simulink model "PID"  (R2021b)
settings: Solver=VariableStepAuto  StartTime=0.0  StopTime=inf  RelTol=1e-3
undefined symbols (not defined in the file or in its folder): K, my_password, recipient, sender, sendMail, T
libraries: slpidlib x2, flexy2_lib x1, dspstat3 x1
settings Model: Creator=timon  LastModifiedBy=marekwadinger

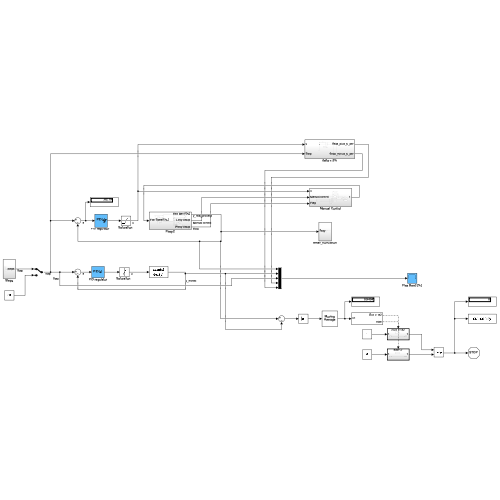
[thumbnail: Simulink's stored preview of the top-level diagram]
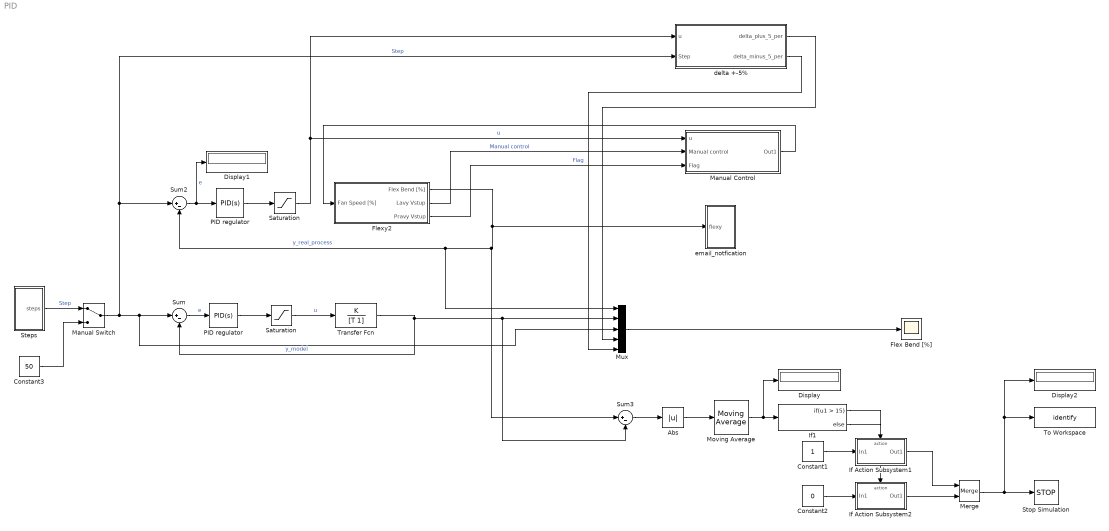
== system PID ==
  Abs : Abs
  Constant1 : Constant
  Constant2 : Constant  Value=0
  Constant3 : Constant  Value=50
  Display : Display
  Display1 : Display
  Display2 : Display
  Flex Bend [%] : Scope
  Flexy2 : Subsystem
  If Action Subsystem1 : Subsystem  TreatAsAtomicUnit=on
  If Action Subsystem2 : Subsystem  TreatAsAtomicUnit=on
  If1 : If  IfExpression=u1 > 15
  Manual Control : Subsystem
  Manual Switch : ManualSwitch
  Merge : Merge
  Moving Average : dspstat3/Moving Average  Method=Sliding window  ForgettingFactorPort=off  SpecifyWindowLength=on  WindowLength=10000  ForgettingFactor=0.9  SimulateUsing=Code generation
  Mux : Mux  Inputs=5
  PID regulator : slpidlib/PID Controller  Controller=PID  Form=Parallel  TimeDomain=Continuous-time  UseExternalTs=off  SampleTime=-1  IntegratorMethod=Forward Euler  FilterMethod=Forward Euler  ControllerParametersSource=internal  P=2.611  I=2.611/0.32485  D=2.611*0.082197  UseFilter=on  N=100  TunerSelectOption=Transfer Function Based (PID Tuner App)  InitialConditionSource=internal  InitialConditionForIntegrator=0  InitialConditionForFilter=0  DifferentiatorICPrevScaledInput=0  ExternalReset=none  TrackingMode=off  Kt=1  LimitOutput=off  SatLimitsSource=internal  UpperSaturationLimit=inf  LowerSaturationLimit=-inf  LinearizeAsGain=on  AntiWindupMode=none  Kb=1  POutMin=[]  POutMax=[]  IOutMin=[]  IOutMax=[]  DOutMin=[]  DOutMax=[]  NOutMin=[]  NOutMax=[]  SumOutMin=[]  SumOutMax=[]  SaturationOutMin=[]  SaturationOutMax=[]  PParamMin=[]  PParamMax=[]  IParamMin=[]  IParamMax=[]  DParamMin=[]  DParamMax=[]  NParamMin=[]  NParamMax=[]  KbParamMin=[]  KbParamMax=[]  KtParamMin=[]  KtParamMax=[]  KbOutMin=[]  KbOutMax=[]  KtOutMin=[]  KtOutMax=[]  IntegratorOutMin=[]  IntegratorOutMax=[]  FilterOutMin=[]  FilterOutMax=[]  SumI1OutMin=[]  SumI1OutMax=[]  SumI2OutMin=[]  SumI2OutMax=[]  SumI3OutMin=[]  SumI3OutMax=[]  SumI4OutMin=[]  SumI4OutMax=[]  SumDOutMin=[]  SumDOutMax=[]  DifferentiatorOutMin=[]  DifferentiatorOutMax=[]  FilterDiffOutCoefMin=[]  FilterDiffOutCoefMax=[]  ReciprocalOutMin=[]  ReciprocalOutMax=[]  SumDenOutMin=[]  SumDenOutMax=[]  SumNumOutMin=[]  SumNumOutMax=[]  DivideOutMin=[]  DivideOutMax=[]  UdiffTsProdOutMin=[]  UdiffTsProdOutMax=[]  NTsProdOutMin=[]  NTsProdOutMax=[]  UintegralTsProdOutMin=[]  UintegralTsProdOutMax=[]  UngainTsProdOutMin=[]  UngainTsProdOutMax=[]  IntegratorContinuousStateAttributes=''  IntegratorStateMustResolveToSignalObject=off  IntegratorRTWStateStorageClass=Auto  FilterContinuousStateAttributes=''  FilterStateMustResolveToSignalObject=off  FilterRTWStateStorageClass=Auto  ParallelPVariant=InternalParameters  IdealPVariant=Disabled  IVariant=InternalParameters  DVariant=InternalParameters  IntegratorVariant=Continuous  SatVariant=Disabled  AWVariant=Passthrough  PCopyVariant=Disabled  TRVariant=Disabled  FdbkBlocksVariant=Forward  IdealPFdbkVariant=Disabled  SatFdbkVariant=Disabled  DerivativeFilterVariant=ContFilter  NVariant=InternalParameters  NCopyVariant=Disabled  FilterICVariant=InternalICsFilter  IntegratorICVariant=InternalICs  ExternalResetVariant=Disabled  TRSumVariant=Passthrough  SumFdbkVariant=Disabled  SumVariant=Sum_PID  TsampFilterVariant=InternalTs  TsampNgainVariant=Passthrough  TsampIntegralVariant=Passthrough  ExternalSaturationOutDataTypeStr=Inherit: Same as second input
  "PID regulator  " : slpidlib/PID Controller  Controller=PID  Form=Parallel  TimeDomain=Continuous-time  UseExternalTs=off  SampleTime=-1  IntegratorMethod=Forward Euler  FilterMethod=Forward Euler  ControllerParametersSource=internal  P=2.611  I=2.611/0.32485  D=2.611*0.082197  UseFilter=on  N=100  TunerSelectOption=Transfer Function Based (PID Tuner App)  InitialConditionSource=internal  InitialConditionForIntegrator=0  InitialConditionForFilter=0  DifferentiatorICPrevScaledInput=0  ExternalReset=none  TrackingMode=off  Kt=1  LimitOutput=on  SatLimitsSource=internal  UpperSaturationLimit=100  LowerSaturationLimit=0  LinearizeAsGain=on  AntiWindupMode=back-calculation  Kb=1  POutMin=[]  POutMax=[]  IOutMin=[]  IOutMax=[]  DOutMin=[]  DOutMax=[]  NOutMin=[]  NOutMax=[]  SumOutMin=[]  SumOutMax=[]  SaturationOutMin=[]  SaturationOutMax=[]  PParamMin=[]  PParamMax=[]  IParamMin=[]  IParamMax=[]  DParamMin=[]  DParamMax=[]  NParamMin=[]  NParamMax=[]  KbParamMin=[]  KbParamMax=[]  KtParamMin=[]  KtParamMax=[]  KbOutMin=[]  KbOutMax=[]  KtOutMin=[]  KtOutMax=[]  IntegratorOutMin=[]  IntegratorOutMax=[]  FilterOutMin=[]  FilterOutMax=[]  SumI1OutMin=[]  SumI1OutMax=[]  SumI2OutMin=[]  SumI2OutMax=[]  SumI3OutMin=[]  SumI3OutMax=[]  SumI4OutMin=[]  SumI4OutMax=[]  SumDOutMin=[]  SumDOutMax=[]  DifferentiatorOutMin=[]  DifferentiatorOutMax=[]  FilterDiffOutCoefMin=[]  FilterDiffOutCoefMax=[]  ReciprocalOutMin=[]  ReciprocalOutMax=[]  SumDenOutMin=[]  SumDenOutMax=[]  SumNumOutMin=[]  SumNumOutMax=[]  DivideOutMin=[]  DivideOutMax=[]  UdiffTsProdOutMin=[]  UdiffTsProdOutMax=[]  NTsProdOutMin=[]  NTsProdOutMax=[]  UintegralTsProdOutMin=[]  UintegralTsProdOutMax=[]  UngainTsProdOutMin=[]  UngainTsProdOutMax=[]  IntegratorContinuousStateAttributes=''  IntegratorStateMustResolveToSignalObject=off  IntegratorRTWStateStorageClass=Auto  FilterContinuousStateAttributes=''  FilterStateMustResolveToSignalObject=off  FilterRTWStateStorageClass=Auto  ParallelPVariant=InternalParameters  IdealPVariant=Disabled  IVariant=InternalParameters  DVariant=InternalParameters  IntegratorVariant=Continuous  SatVariant=Enabled  AWVariant=BackCalculation  PCopyVariant=Disabled  TRVariant=Disabled  FdbkBlocksVariant=Forward  IdealPFdbkVariant=Disabled  SatFdbkVariant=Disabled  DerivativeFilterVariant=ContFilter  NVariant=InternalParameters  NCopyVariant=Disabled  FilterICVariant=InternalICsFilter  IntegratorICVariant=InternalICs  ExternalResetVariant=Disabled  TRSumVariant=Passthrough  SumFdbkVariant=Disabled  SumVariant=Sum_PID  TsampFilterVariant=InternalTs  TsampNgainVariant=Passthrough  TsampIntegralVariant=Passthrough  ExternalSaturationOutDataTypeStr=Inherit: Same as second input
  "Saturation " : Saturate  UpperLimit=100  LowerLimit=0
  "Saturation  " : Saturate  UpperLimit=100  LowerLimit=0
  Steps : Subsystem
  Stop Simulation : Stop
  Sum : Sum  Inputs=|+-
  Sum2 : Sum  Inputs=|+-
  Sum3 : Sum  Inputs=|+-
  To Workspace : ToWorkspace  VariableName=identify  SaveFormat=Timeseries  SampleTime=-1
      settings: MaxDataPoints=1
  Transfer Fcn : TransferFcn  Numerator=K  Denominator=[T 1]
  delta +-5% : Subsystem
  email_notfication : Subsystem
  wires:
  Manual Switch/1 -> delta +-5%/2(Step), Sum2/1, Mux/3, Sum/1  "Step"
  "Saturation  "/1 -> Transfer Fcn/1  "u"
  PID regulator/1 -> "Saturation  "/1
  Sum/1 -> PID regulator/1  "e"
  Mux/1 -> Flex Bend [%]/1
  Transfer Fcn/1 -> Sum/2, Sum3/2, Mux/2  "y_model"
  Sum2/1 -> Display1/1, "PID regulator  "/1  "e"
  Flexy2/1(Flex Bend [%]) -> Sum3/1, Sum2/2, Mux/1, email_notfication/1(flexy)  "y_real_process"
  "PID regulator  "/1 -> "Saturation "/1
  "Saturation "/1 -> delta +-5%/1(u), Manual Control/1(u)  "u"
  Flexy2/2(Lavy Vstup) -> Manual Control/2(Manual control)  "Manual control"
  Flexy2/3(Pravy Vstup) -> Manual Control/3(Flag)  "Flag"
  Manual Control/1(Out1) -> Flexy2/1(Fan Speed [%])
  delta +-5%/1(delta_plus_5_per) -> Mux/4
  delta +-5%/2(delta_minus_5_per) -> Mux/5
  Sum3/1 -> Abs/1
  Abs/1 -> Moving Average/1
  If1/2 -> If Action Subsystem2/Action
  If Action Subsystem1/1(Out1) -> Merge/1
  Constant2/1 -> If Action Subsystem2/1(In1)
  If Action Subsystem2/1(Out1) -> Merge/2
  Constant1/1 -> If Action Subsystem1/1(In1)
  If1/1 -> If Action Subsystem1/Action
  Moving Average/1 -> If1/1, Display/1
  Merge/1 -> To Workspace/1, Display2/1, Stop Simulation/1
  Steps/1(steps) -> Manual Switch/1  "Step"
  Constant3/1 -> Manual Switch/2

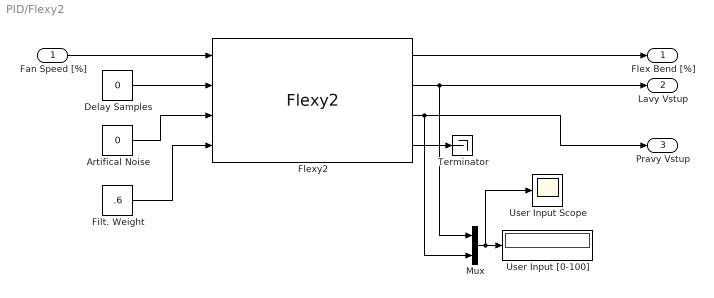
== system PID/Flexy2 ==
  Fan Speed [%] : Inport
  Artifical Noise : Constant  Value=0
  Delay Samples : Constant  Value=0
  Filt. Weight : Constant  Value=.6
  Flexy2 : flexy2_lib/Flexy2  SystemSampleTime=-1  VariantActivationTime=update diagram  Latency=0  AutoFrameSizeCalculation=off
  Mux : Mux  Inputs=2
  Terminator : Terminator
  User Input Scope : Scope
  User Input [0-100] : Display
  Flex Bend [%] : Outport
  Lavy Vstup : Outport  Port=2
  Pravy Vstup : Outport  Port=3
  wires:
  Fan Speed [%]/1 -> Flexy2/1
  Delay Samples/1 -> Flexy2/2
  Flexy2/2 -> Mux/1, Lavy Vstup/1
  Filt. Weight/1 -> Flexy2/4
  Flexy2/1 -> Flex Bend [%]/1
  Mux/1 -> User Input Scope/1, User Input [0-100]/1
  Flexy2/4 -> Terminator/1
  Flexy2/3 -> Mux/2, Pravy Vstup/1
  Artifical Noise/1 -> Flexy2/3

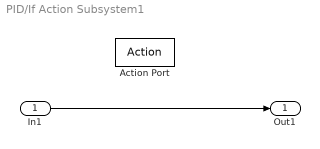
== system PID/If Action Subsystem1 ==
  In1 : Inport
  Action Port : ActionPort  ActionPortLabel=if(u1 > 15)
  Out1 : Outport
  wires:
  In1/1 -> Out1/1

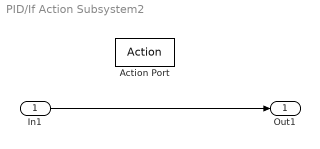
== system PID/If Action Subsystem2 ==
  In1 : Inport
  Action Port : ActionPort  ActionPortLabel=else
  Out1 : Outport
  wires:
  In1/1 -> Out1/1

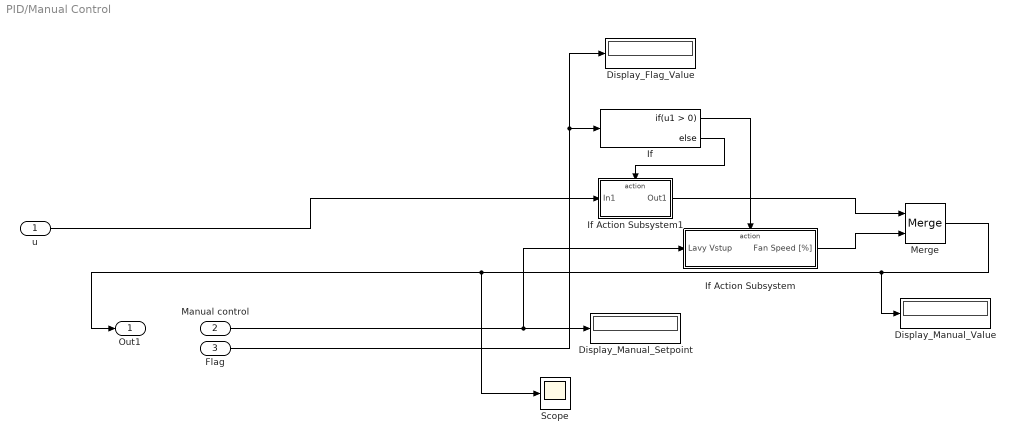
== system PID/Manual Control ==
  u : Inport
  Manual control : Inport  Port=2
  Flag : Inport  Port=3
  Display_Flag_Value : Display
  Display_Manual_Setpoint : Display
  Display_Manual_Value : Display
  If : If
  If Action Subsystem : Subsystem  TreatAsAtomicUnit=on
  If Action Subsystem1 : Subsystem  TreatAsAtomicUnit=on
  Merge : Merge
  Scope : Scope
  Out1 : Outport
  wires:
  If/2 -> If Action Subsystem1/Action
  If Action Subsystem/1(Fan Speed [%]) -> Merge/2
  Merge/1 -> Display_Manual_Value/1, Out1/1, Scope/1
  If/1 -> If Action Subsystem/Action
  If Action Subsystem1/1(Out1) -> Merge/1
  Flag/1 -> Display_Flag_Value/1, If/1
  Manual control/1 -> If Action Subsystem/1(Lavy Vstup), Display_Manual_Setpoint/1
  u/1 -> If Action Subsystem1/1(In1)

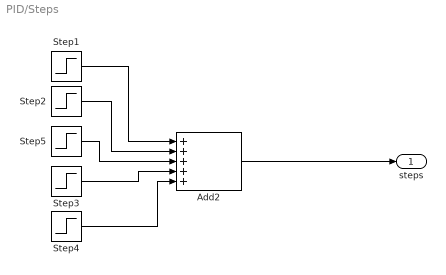
== system PID/Steps ==
  Add2 : Sum  Inputs=+++++
  Step1 : Step  Time=20  Before=30  After=1.1*50  SampleTime=0
  Step2 : Step  Time=40  After=0.2*50  SampleTime=0
  Step3 : Step  Time=80  After=0.7*50  SampleTime=0
  Step4 : Step  Time=100  After=-0.6*50  SampleTime=0
  Step5 : Step  Time=60  After=-0.5*50  SampleTime=0
  steps : Outport
  wires:
  Add2/1 -> steps/1
  Step1/1 -> Add2/1
  Step5/1 -> Add2/3
  Step2/1 -> Add2/2
  Step3/1 -> Add2/4
  Step4/1 -> Add2/5

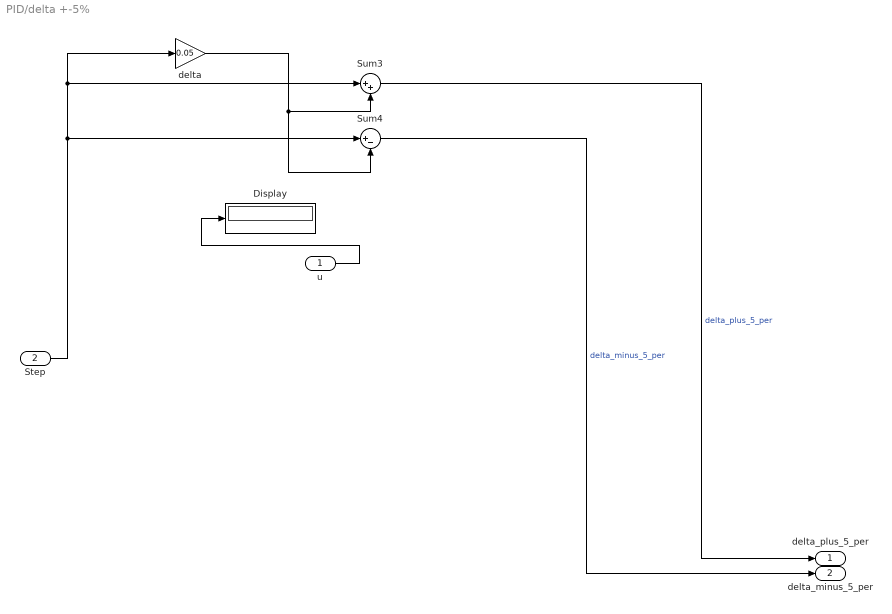
== system PID/delta +-5% ==
  u : Inport
  Step : Inport  Port=2
  Display : Display
  Sum3 : Sum  Inputs=|++
  Sum4 : Sum  Inputs=|+-
  delta : Gain  Gain=0.05
  delta_plus_5_per : Outport
  delta_minus_5_per : Outport  Port=2
  wires:
  delta/1 -> Sum4/2, Sum3/2
  u/1 -> Display/1
  Step/1 -> Sum3/1, delta/1, Sum4/1
  Sum3/1 -> delta_plus_5_per/1  "delta_plus_5_per"
  Sum4/1 -> delta_minus_5_per/1  "delta_minus_5_per"

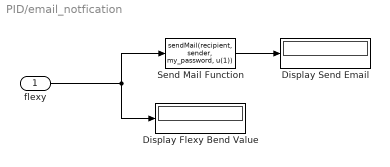
== system PID/email_notfication ==
  flexy : Inport
  Display Flexy Bend Value : Display
  Display Send Email : Display
  Send Mail Function : MATLABFcn  MATLABFcn=sendMail(recipient, sender, my_password, u(1))
  wires:
  flexy/1 -> Display Flexy Bend Value/1, Send Mail Function/1
  Send Mail Function/1 -> Display Send Email/1

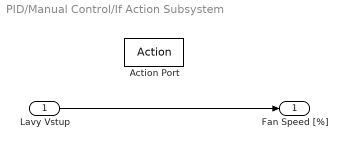
== system PID/Manual Control/If Action Subsystem ==
  Lavy Vstup : Inport
  Action Port : ActionPort  ActionPortLabel=if(u1 > 0)
  Fan Speed [%] : Outport
  wires:
  Lavy Vstup/1 -> Fan Speed [%]/1

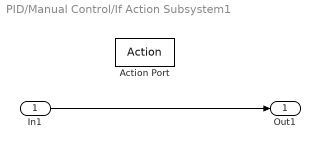
== system PID/Manual Control/If Action Subsystem1 ==
  In1 : Inport
  Action Port : ActionPort  ActionPortLabel=else
  Out1 : Outport
  wires:
  In1/1 -> Out1/1
